simulink model "liaisonCDMA2"  (R2012b)
settings: Solver=ode45  StartTime=0.0  StopTime=10.0  RelTol=1e-3
undefined symbols (not defined in the file or in its folder): Fs, get, sided, Two
libraries: dspsnks4 x12, commsink2 x3, commseqgen2 x3, commfilt2 x3, commrandsrc2 x3, dspsigops x3, commutil2 x3
settings Model: Creator=mcaceres  LastModifiedBy=mcaceres

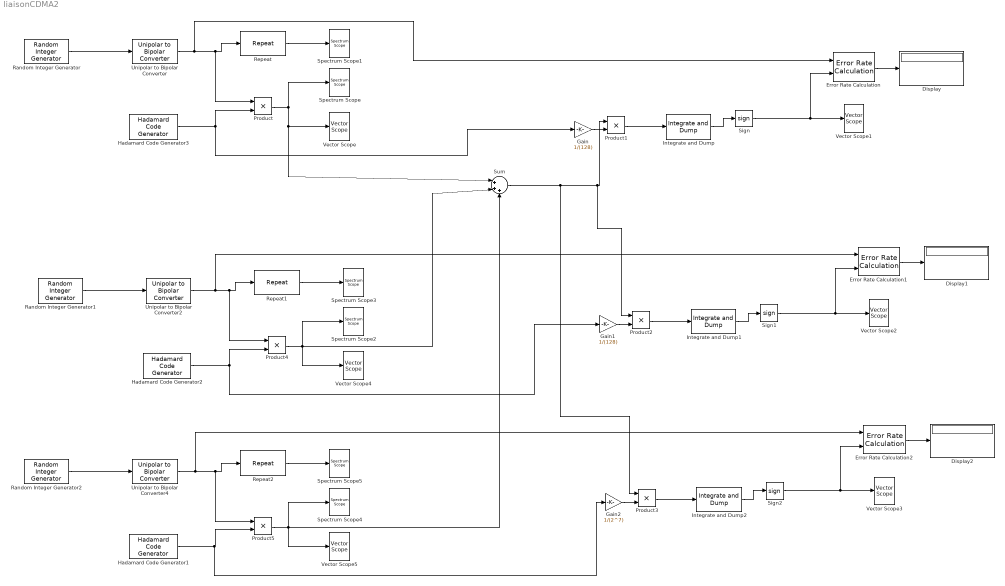
== system liaisonCDMA2 ==
  Display : Display
  Display1 : Display
  Display2 : Display
  Error Rate Calculation : commsink2/Error Rate Calculation  N=1  st_delay=0  cp_mode=Entire frame  subframe=[]  PMode=Port  WsName=ErrorVec  RsMode2=off  stop=off  numErr=100  maxBits=1e6
  Error Rate Calculation1 : commsink2/Error Rate Calculation  N=1  st_delay=0  cp_mode=Entire frame  subframe=[]  PMode=Port  WsName=ErrorVec  RsMode2=off  stop=off  numErr=100  maxBits=1e6
  Error Rate Calculation2 : commsink2/Error Rate Calculation  N=1  st_delay=0  cp_mode=Entire frame  subframe=[]  PMode=Port  WsName=ErrorVec  RsMode2=off  stop=off  numErr=100  maxBits=1e6
  Gain : Gain  Gain=1/(128)
  Gain1 : Gain  Gain=1/(128)
  Gain2 : Gain  Gain=1/(2^7)
  Hadamard Code Generator1 : commseqgen2/Hadamard Code Generator  length=128  index=50  ts=10^-6/128  frameBased=off  sampPerFrame=128  outDataType=double
  Hadamard Code Generator2 : commseqgen2/Hadamard Code Generator  length=128  index=44  ts=10^-6/128  frameBased=off  sampPerFrame=128  outDataType=double
  Hadamard Code Generator3 : commseqgen2/Hadamard Code Generator  length=128  index=47  ts=10^-6/128  frameBased=off  sampPerFrame=128  outDataType=double
  Integrate and Dump : commfilt2/Integrate and Dump  obssamples=128  offsetsamples=0  nodump=off  roundingMode=Floor  overflowMode=off
  Integrate and Dump1 : commfilt2/Integrate and Dump  obssamples=128  offsetsamples=0  nodump=off  roundingMode=Floor  overflowMode=off
  Integrate and Dump2 : commfilt2/Integrate and Dump  obssamples=128  offsetsamples=0  nodump=off  roundingMode=Floor  overflowMode=off
  Product{,1..5} (6 alike) : Product  RndMeth=Zero
  Random Integer Generator : commrandsrc2/Random Integer Generator  mul=2  seed=37  Ts=10^-6  frameBased=off  sampPerFrame=1  orient=off  outDataType=double
  Random Integer Generator1 : commrandsrc2/Random Integer Generator  mul=2  seed=14  Ts=10^-6  frameBased=off  sampPerFrame=1  orient=off  outDataType=double
  Random Integer Generator2 : commrandsrc2/Random Integer Generator  mul=2  seed=41  Ts=10^-6  frameBased=off  sampPerFrame=1  orient=off  outDataType=double
  Repeat : dspsigops/Repeat  N=2^6-1  InputProcessing=Columns as channels (frame based)  RateOptions=Allow multirate processing  ic=0  mode=Unused parameter value
  Repeat1 : dspsigops/Repeat  N=2^6-1  InputProcessing=Columns as channels (frame based)  RateOptions=Allow multirate processing  ic=0  mode=Unused parameter value
  Repeat2 : dspsigops/Repeat  N=2^6-1  InputProcessing=Columns as channels (frame based)  RateOptions=Allow multirate processing  ic=0  mode=Unused parameter value
  Sign : Signum  ZeroCross=off
  Sign1 : Signum  ZeroCross=off
  Sign2 : Signum  ZeroCross=off
  Spectrum Scope{,1..5} (6 alike) : dspsnks4/Spectrum Scope  ScopeProperties=on  Domain=Frequency  HorizSpan=1  UseBuffer=on  BufferSize=128  Overlap=0  TreatMby1Signals=One channel  inpFftLenInherit=on  FFTlength=128  numAvg=20  DisplayProperties=off  AxisGrid=on  Memory=off  FrameNumber=on  AxisLegend=off  AxisZoom=off  OpenScopeAtSimStart=on  OpenScopeImmediately=off  FigPos=get(0,'defaultfigureposition')  AxisProperties=off  XUnits=Hertz  XRange=Two-sided ((-Fs/2...Fs/2])  XDisplay=0  InheritXIncr=on  XIncr=1.0  XLabel=Samples  XLimit=Auto  YUnits=dBW/Hertz  XMax=1  XMin=0  YLabel=Magnitude-squared, dB  LineProperties=off  wintypeSpecScope=Hann  RsSpecScope=50  betaSpecScope=5  winsampSpecScope=Periodic  XAxisParamsVer=6.9  isFrameUpgraded=on
      settings: YMin=-10  YMax=10
  Sum : Sum  Inputs=|+++
  Unipolar to Bipolar Converter : commutil2/Unipolar to Bipolar Converter  M=2  polarity=Positive  dataType=Inherit via internal rule
  Unipolar to Bipolar Converter2 : commutil2/Unipolar to Bipolar Converter  M=2  polarity=Positive  dataType=Inherit via internal rule
  Unipolar to Bipolar Converter4 : commutil2/Unipolar to Bipolar Converter  M=2  polarity=Positive  dataType=Inherit via internal rule
  Vector Scope : dspsnks4/Vector Scope  ScopeProperties=on  Domain=Time  HorizSpan=3*((2^6)-1)  DisplayProperties=off  AxisGrid=on  Memory=off  FrameNumber=on  AxisLegend=off  AxisZoom=off  OpenScopeAtSimStart=on  OpenScopeImmediately=off  FigPos=get(0,'defaultfigureposition')  AxisProperties=off  XUnits=Hertz  XRange=[0...Fs/2]  InheritXIncr=on  XIncr=1  XLabel=Time  XLimit=Auto  XMin=0  XMax=1  XStart=0  YUnits=dB  YLabel=Amplitude  LineProperties=off  LineStyles=None  LineMarkers=o  XAxisParamsVer=6.9
      settings: YMin=-10  YMax=10
  Vector Scope1 : dspsnks4/Vector Scope  ScopeProperties=on  Domain=Time  HorizSpan=3*((2^6)-1)  DisplayProperties=off  AxisGrid=on  Memory=off  FrameNumber=on  AxisLegend=off  AxisZoom=off  OpenScopeAtSimStart=on  OpenScopeImmediately=off  FigPos=get(0,'defaultfigureposition')  AxisProperties=off  XUnits=Hertz  XRange=[0...Fs/2]  InheritXIncr=on  XIncr=1  XLabel=Time  XLimit=Auto  XMin=0  XMax=1  XStart=0  YUnits=dB  YLabel=Amplitude  LineProperties=off  LineStyles=None  LineMarkers=o  LineColors=b  XAxisParamsVer=6.9
      settings: YMin=-10  YMax=10
  Vector Scope2 : dspsnks4/Vector Scope  ScopeProperties=on  Domain=Time  HorizSpan=3*((2^6)-1)  DisplayProperties=off  AxisGrid=on  Memory=off  FrameNumber=on  AxisLegend=off  AxisZoom=off  OpenScopeAtSimStart=on  OpenScopeImmediately=off  FigPos=get(0,'defaultfigureposition')  AxisProperties=off  XUnits=Hertz  XRange=[0...Fs/2]  InheritXIncr=on  XIncr=1  XLabel=Time  XLimit=Auto  XMin=0  XMax=1  XStart=0  YUnits=dB  YLabel=Amplitude  LineProperties=off  LineStyles=None  LineMarkers=o  LineColors=b  XAxisParamsVer=6.9
      settings: YMin=-10  YMax=10
  Vector Scope3 : dspsnks4/Vector Scope  ScopeProperties=on  Domain=Time  HorizSpan=3*((2^6)-1)  DisplayProperties=off  AxisGrid=on  Memory=off  FrameNumber=on  AxisLegend=off  AxisZoom=off  OpenScopeAtSimStart=on  OpenScopeImmediately=off  FigPos=get(0,'defaultfigureposition')  AxisProperties=off  XUnits=Hertz  XRange=[0...Fs/2]  InheritXIncr=on  XIncr=1  XLabel=Time  XLimit=Auto  XMin=0  XMax=1  XStart=0  YUnits=dB  YLabel=Amplitude  LineProperties=off  LineStyles=None  LineMarkers=o  LineColors=b  XAxisParamsVer=6.9
      settings: YMin=-10  YMax=10
  Vector Scope4 : dspsnks4/Vector Scope  ScopeProperties=on  Domain=Time  HorizSpan=3*((2^6)-1)  DisplayProperties=off  AxisGrid=on  Memory=off  FrameNumber=on  AxisLegend=off  AxisZoom=off  OpenScopeAtSimStart=on  OpenScopeImmediately=off  FigPos=get(0,'defaultfigureposition')  AxisProperties=off  XUnits=Hertz  XRange=[0...Fs/2]  InheritXIncr=on  XIncr=1  XLabel=Time  XLimit=Auto  XMin=0  XMax=1  XStart=0  YUnits=dB  YLabel=Amplitude  LineProperties=off  LineStyles=None  LineMarkers=o  XAxisParamsVer=6.9
      settings: YMin=-10  YMax=10
  Vector Scope5 : dspsnks4/Vector Scope  ScopeProperties=on  Domain=Time  HorizSpan=3*((2^6)-1)  DisplayProperties=off  AxisGrid=on  Memory=off  FrameNumber=on  AxisLegend=off  AxisZoom=off  OpenScopeAtSimStart=on  OpenScopeImmediately=off  FigPos=get(0,'defaultfigureposition')  AxisProperties=off  XUnits=Hertz  XRange=[0...Fs/2]  InheritXIncr=on  XIncr=1  XLabel=Time  XLimit=Auto  XMin=0  XMax=1  XStart=0  YUnits=dB  YLabel=Amplitude  LineProperties=off  LineStyles=None  LineMarkers=o  XAxisParamsVer=6.9
      settings: YMin=-10  YMax=10
  wires:
  Integrate and Dump/1 -> Sign/1
  Error Rate Calculation/1 -> Display/1
  Sign/1 -> Error Rate Calculation/2, Vector Scope1/1
  Gain/1 -> Product1/2
  Product1/1 -> Integrate and Dump/1
  Product/1 -> Sum/1, Vector Scope/1, Spectrum Scope/1
  Unipolar to Bipolar Converter/1 -> Error Rate Calculation/1, Repeat/1, Product/1
  Random Integer Generator/1 -> Unipolar to Bipolar Converter/1
  Repeat/1 -> Spectrum Scope1/1
  Hadamard Code Generator3/1 -> Gain/1, Product/2
  Sum/1 -> Product3/1, Product2/1, Product1/1
  Integrate and Dump1/1 -> Sign1/1
  Error Rate Calculation1/1 -> Display1/1
  Sign1/1 -> Error Rate Calculation1/2, Vector Scope2/1
  Gain1/1 -> Product2/2
  Product2/1 -> Integrate and Dump1/1
  Integrate and Dump2/1 -> Sign2/1
  Error Rate Calculation2/1 -> Display2/1
  Sign2/1 -> Error Rate Calculation2/2, Vector Scope3/1
  Gain2/1 -> Product3/2
  Product3/1 -> Integrate and Dump2/1
  Product4/1 -> Sum/2, Vector Scope4/1, Spectrum Scope2/1
  Unipolar to Bipolar Converter2/1 -> Error Rate Calculation1/1, Repeat1/1, Product4/1
  Random Integer Generator1/1 -> Unipolar to Bipolar Converter2/1
  Repeat1/1 -> Spectrum Scope3/1
  Hadamard Code Generator2/1 -> Gain1/1, Product4/2
  Product5/1 -> Sum/3, Vector Scope5/1, Spectrum Scope4/1
  Unipolar to Bipolar Converter4/1 -> Error Rate Calculation2/1, Repeat2/1, Product5/1
  Random Integer Generator2/1 -> Unipolar to Bipolar Converter4/1
  Repeat2/1 -> Spectrum Scope5/1
  Hadamard Code Generator1/1 -> Gain2/1, Product5/2
